simulink model "L2_Q4_Sim"  (R2015a)
settings: Solver=ode3  StartTime=0.0  StopTime=tf  FixedStep=t_step  RelTol=1e-3
values from neighbouring files (symbols this model uses):
  c = 2*(rand-0.5)    [L2_Q4.m]
  K = 200    [L2_Q4.m]
  k = 6*rand-1    [L2_Q4.m]
  lamb = 1    [L2_Q4.m]
  phi = 0.1    [L2_Q4.m]
  xd1 = 5    [L2_Q2.m]    (also in L2_Q4.m)
settings Model: Creator=Marcelo  LastModifiedBy=Marcelo

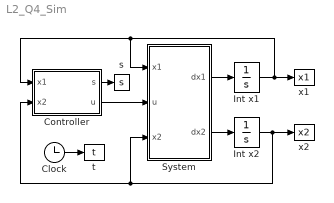
== system L2_Q4_Sim ==
  Clock : Clock
  Controller : MATLAB Function  TreatAsAtomicUnit=on
  Int x1 : Integrator
  Int x2 : Integrator
  System : MATLAB Function  TreatAsAtomicUnit=on
  s : ToWorkspace  VariableName=s  SampleTime=-1
  t : ToWorkspace  VariableName=t  SampleTime=-1
  x1 : ToWorkspace  VariableName=x1  SampleTime=-1
  x2 : ToWorkspace  VariableName=x2  SampleTime=-1
  wires:
  Clock/1 -> t/1
  Int x2/1 -> Controller/2(x2), System/3(x2), x2/1
  Int x1/1 -> System/1(x1), Controller/1(x1), x1/1
  System/2(dx2) -> Int x2/1
  System/1(dx1) -> Int x1/1
  Controller/2(u) -> System/2(u)
  Controller/1(s) -> s/1

== matlab function L2_Q4_Sim/System ==
  data: x1 input; u input; dx1 output; dx2 output; x2 input; c parameter; k parameter
function [dx1, dx2] = fcn(x1, u, x2, c, k)
dx1 = x2;
dx2 = u - c*abs(x1)*x2^2 - k*x1^3*cos(2*x1);

== matlab function L2_Q4_Sim/Controller ==
  data: s output; u output; x1 input; x2 input; xd1 parameter; lamb parameter; phi parameter; K parameter
function [s,u] = fcn(x1, x2, xd1, lamb, phi, K)
u_hat = 2*x1^3*cos(2*x1) - lamb*x2;
s = x2 + lamb * (x1 - xd1);
sat_s = min(1, max(-1, s/phi));
u = u_hat - K * sat_s;
